simulink library "motohawk_engine_lib"  (Simulink 6.3)
undefined symbols (not defined in the file or in its folder): cast_val, IndPowerMax, InjSequence, lookup_group, MAF_Sensor_p, motohawk_tex, motohawk_vardec_config_group, motohawk_vardec_path, SampleTime, SparkSequence, SteadyStateECT, txtTitle, WarmUpTimeConst
libraries: MotoHawk_lib x234, motohawk_annotations_lib x22, motohawk_control_primitives_lib x20, motohawk_engine_lib x8, motohawk_control_primitives_lib_new x3
(part 2 of 7)

== system motohawk_engine_lib/Analog Switch ==
  ADC : Inport
  0 = No Inversion 1 = Inversion : MotoHawk_lib/Calibration & Probing Blocks/motohawk_calibration  nam=[prefix 'Polarity']  val=boolean(polarity-1)  storage=Calibration  show_more=on  name_source=Use Parameter  data_type=Inherit from 'Default Value'  read_level=1  write_level=1  ovr_cals=on  view_as=Number  enum_struct={'Disabled', 'Enabled'}  vector_style=Wide Row  use_help_units=on  help="'0 = High True    1 = Low True'"  units='bool'  use_header_enum=off  row_header_enum={}  col_header_enum={}  use_min_max=off  min_val=-inf  max_val=inf  use_precision=off  precision=''  gain=1  offset=0  exp=1  use_mototune_group=on  mototune_group=[group ' | ' nam ' Config']
  Data Type Conversion : DataTypeConversion  SaturateOnIntegerOverflow=on  RndMeth=Zero
  Logical Operator : Logic  Operator=XOR
  Override in Engineering Units : MotoHawk_lib/Calibration & Probing Blocks/motohawk_override_abs  parent_name=nam  show_more=on  name_source=Use Parameter  parent_read_level=1  parent_override_level=1  view_as=Number  enum_struct={'Disabled', 'Enabled'}  use_help_units=on  parent_help='Override actuator, in engineering units'  parent_units='Boolean'  use_min_max=off  parent_min=-inf  parent_max=inf  use_precision=off  parent_precision=''  parent_gain=1  parent_offset=0  parent_exp=1  use_mototune_group=on  parent_group=group
  Relational Operator : RelationalOperator  Operator=>
  SwitchPoint : MotoHawk_lib/Calibration & Probing Blocks/motohawk_calibration  nam=[prefix 'SwitchPt']  val=switchpoint  storage=Calibration  show_more=on  name_source=Use Parameter  data_type=Inherit from 'Default Value'  read_level=1  write_level=1  ovr_cals=on  view_as=Number  enum_struct={'Disabled', 'Enabled'}  vector_style=Wide Row  use_help_units=on  help='Defines switch point in ADC units boolean conversion'  units='ADC'  use_header_enum=off  row_header_enum={}  col_header_enum={}  use_min_max=off  min_val=-inf  max_val=inf  use_precision=off  precision=''  gain=1  offset=0  exp=1  use_mototune_group=on  mototune_group=[group ' | ' nam ' Config']
  motohawk_probe : MotoHawk_lib/Calibration & Probing Blocks/motohawk_probe  nam=nam  show_more=on  name_source=Use Parameter  read_level=1  view_as=Number  enum_struct={'Disabled', 'Enabled'}  vector_style=Wide Row  use_help_units=on  help='Display output in engineering units'  units='Boolean'  use_header_enum=off  row_header_enum={}  col_header_enum={}  use_precision=off  precision=''  gain=1  offset=0  exp=1  use_mototune_group=on  mototune_group=group
  motohawk_probe1 : MotoHawk_lib/Calibration & Probing Blocks/motohawk_probe  nam=[nam '_Raw']  show_more=on  name_source=Use Parameter  read_level=1  view_as=Number  enum_struct={'Disabled', 'Enabled'}  vector_style=Wide Row  use_help_units=on  help='Display output in engineering units'  units='ADC'  use_header_enum=off  row_header_enum={}  col_header_enum={}  use_precision=off  precision=''  gain=1  offset=0  exp=1  use_mototune_group=on  mototune_group=group
  DiscOut : Outport
  wires:
  ADC/1 -> Data Type Conversion/1
  0 = No Inversion 1 = Inversion/1 -> Logical Operator/2
  Logical Operator/1 -> Override in Engineering Units/1
  Relational Operator/1 -> Logical Operator/1
  SwitchPoint/1 -> Relational Operator/2
  Override in Engineering Units/1 -> DiscOut/1, motohawk_probe/1
  Data Type Conversion/1 -> Relational Operator/1, motohawk_probe1/1

== system motohawk_engine_lib/Analog Switch1 ==
  Boolean : Inport
  0 = No Inversion 1 = Inversion : MotoHawk_lib/Calibration & Probing Blocks/motohawk_calibration  nam=[prefix 'Polarity']  val=boolean(polarity-1)  storage=Calibration  show_more=on  name_source=Use Parameter  data_type=Inherit from 'Default Value'  read_level=1  write_level=1  ovr_cals=on  view_as=Number  enum_struct={'Disabled', 'Enabled'}  vector_style=Wide Row  use_help_units=on  help="'0 = High True    1 = Low True'"  units='bool'  use_header_enum=off  row_header_enum={}  col_header_enum={}  use_min_max=off  min_val=-inf  max_val=inf  use_precision=off  precision=''  gain=1  offset=0  exp=1  use_mototune_group=on  mototune_group=[group ' | ' nam ' Config']
  Logical Operator : Logic  Operator=XOR
  Override in Engineering Units : MotoHawk_lib/Calibration & Probing Blocks/motohawk_override_abs  parent_name=nam  show_more=on  name_source=Use Parameter  parent_read_level=1  parent_override_level=1  view_as=Number  enum_struct={'Disabled', 'Enabled'}  use_help_units=on  parent_help='Override actuator, in engineering units'  parent_units='Boolean'  use_min_max=off  parent_min=-inf  parent_max=inf  use_precision=off  parent_precision=''  parent_gain=1  parent_offset=0  parent_exp=1  use_mototune_group=on  parent_group=group
  motohawk_probe : MotoHawk_lib/Calibration & Probing Blocks/motohawk_probe  nam=nam  show_more=on  name_source=Use Parameter  read_level=1  view_as=Number  enum_struct={'Disabled', 'Enabled'}  vector_style=Wide Row  use_help_units=on  help='Display output in engineering units'  units='Boolean'  use_header_enum=off  row_header_enum={}  col_header_enum={}  use_precision=off  precision=''  gain=1  offset=0  exp=1  use_mototune_group=on  mototune_group=group
  motohawk_probe1 : MotoHawk_lib/Calibration & Probing Blocks/motohawk_probe  nam=[nam '_Raw']  show_more=on  name_source=Use Parameter  read_level=1  view_as=Number  enum_struct={'Disabled', 'Enabled'}  vector_style=Wide Row  use_help_units=on  help='Display output in engineering units'  units='Boolean'  use_header_enum=off  row_header_enum={}  col_header_enum={}  use_precision=off  precision=''  gain=1  offset=0  exp=1  use_mototune_group=on  mototune_group=group
  DiscOut : Outport
  wires:
  Override in Engineering Units/1 -> motohawk_probe/1, DiscOut/1
  Logical Operator/1 -> Override in Engineering Units/1
  0 = No Inversion 1 = Inversion/1 -> Logical Operator/2
  Boolean/1 -> Logical Operator/1, motohawk_probe1/1

== system motohawk_engine_lib/Capture Signal At Startup ==
  note: Count up to "BARO_Count" samples
  Signal_In : Inport
  Enable : EnablePort
  Add : Sum  OutScaling=2^-10
  Add1 : Sum  Inputs=+-  OutScaling=2^-10
  Collect Average : Subsystem
  Constant : Constant  Value=int8(1)  SampleTime=-1
  Logical Operator : Logic  AllPortsSameDT=off  OutDataTypeMode=Boolean
  Relational Operator : RelationalOperator  Operator=<=
  Relational Operator1 : RelationalOperator  Operator=>
  Sum : Sum  Inputs=++|  InputSameDT=on
  Switch : Switch  Threshold=1  ZeroCross=off  InputSameDT=on
  TwoSampleBuffer ToIgnore : Constant  Value=2  SampleTime=-1
  Unit Delay : UnitDelay  Orientation=left  SampleTime=-1
  motohawk_TitleBlock : motohawk_annotations_lib/motohawk_TitleBlock  BlockType_='Mototron_Title_Block'  ttl='Capture Signal At Key Up\newline\rmAverage the first \bfCount\rm samples of the signal on startup, before locking value.'  copyright="'THE INFORMATION CONTAINED IN THIS\\newlineDRAWING IS THE SOLE PROPERTY OF\\newlineMOTOTRON.  ANY REPRODUCTION IN\\newline PART OR AS A WHOLE WITHOUT THE\\newlineWRITTEN PERMISSION OF MOTOTRON\\newline IS PROHIBITED.\\fontsize{16}\\rm\\copyright\\rm\\fontsize{10} 2005'"  address='\fontsize{22}\it\fontname{Arial Black}MotoTron Corporation \fontname{Arial}\fontsize{10}\newline505 Marion Road, Oshkosh, WI, 54901\newlinewww.mototron.com (734) 822-7700'  image_file='mh.jpg'  pretty_print=on  edit_text="strrep([get_param(bdroot, 'Description')  '\\rm\\newline'  get_param(gcs, 'Name')], '_', '\\_')"  edit_as=255
  motohawk_calibration : MotoHawk_lib/Calibration & Probing Blocks/motohawk_calibration  nam=[nam '_Count']  val=int8(count)  storage=Calibration  show_more=on  name_source=Use Parameter  data_type=Inherit from 'Default Value'  read_level=1  write_level=1  ovr_cals=on  view_as=Number  enum_struct={'Disabled', 'Enabled'}  vector_style=Wide Row  use_help_units=on  help='Number of samples to average at key-up to produce signal value'  units=''  use_header_enum=off  row_header_enum={}  col_header_enum={}  use_min_max=off  min_val=-inf  max_val=inf  use_precision=off  precision=''  gain=1  offset=0  exp=1  use_mototune_group=on  mototune_group=grp
  motohawk_override_rel : MotoHawk_lib/Calibration & Probing Blocks/motohawk_override_rel  parent_name=nam  show_more=on  name_source=Use Parameter  parent_read_level=1  parent_override_level=1  use_help_units=on  parent_help='Provides an override to the input by adding this amount to either the locked or running value'  parent_units=units  use_min_max=off  parent_min=-inf  parent_max=inf  use_precision=off  parent_precision=''  parent_gain=1  parent_offset=0  parent_exp=1  use_mototune_group=on  parent_group=grp
  motohawk_probe : MotoHawk_lib/Calibration & Probing Blocks/motohawk_probe  nam=nam  show_more=on  name_source=Use Parameter  read_level=1  view_as=Number  enum_struct={'Disabled', 'Enabled'}  vector_style=Wide Row  use_help_units=on  help=''  units=units  use_header_enum=off  row_header_enum={}  col_header_enum={}  use_precision=off  precision=''  gain=1  offset=0  exp=1  use_mototune_group=on  mototune_group=grp
  Signal_KeyUp : Outport
  wires:
  Add1/1 -> Collect Average/1(Count)
  Relational Operator1/1 -> Logical Operator/2
  Logical Operator/1 -> Collect Average/Enable
  TwoSampleBuffer ToIgnore/1 -> Add1/2, Relational Operator1/2, Add/2
  Add/1 -> Switch/3, Relational Operator/2
  motohawk_calibration/1 -> Add/1
  motohawk_override_rel/1 -> Signal_KeyUp/1, motohawk_probe/1
  Constant/1 -> Sum/2
  Unit Delay/1 -> Sum/1
  Signal_In/1 -> Collect Average/2(Signal)
  Collect Average/1(Captured_Signal) -> motohawk_override_rel/1
  Switch/1 -> Add1/1, Unit Delay/1
  Relational Operator/1 -> Logical Operator/1, Switch/2
  Sum/1 -> Relational Operator1/1, Relational Operator/1, Switch/1

== system motohawk_engine_lib/Closed-Loop O2 Control - Dual Bank ==
  DesEquivRatio : Inport
  O2A [ratio] : Inport  Port=2
  O2B [ratio] : Inport  Port=3
  IndWork [kJ] : Inport  Port=4
  ClosedLoopEnable : Inport  Port=5
  Bus Creator : BusCreator  Inputs=3
  Map O2 Sensors to V8 Cylinders : Subsystem
      mask Display: disp('');
  Multiport Switch : MultiPortSwitch  Inputs=2  zeroidx=on  SaturateOnIntegerOverflow=on  InputSameDT=on
  No Multiplier When Disabled : Constant
  O2 Control State Determination : Subsystem
  O2A : motohawk_engine_lib/O2A  bank=A  display_group=lookup_group(gcb, 'O2Display')  cal_group=lookup_group(gcb, 'O2BankA')
  O2B : motohawk_engine_lib/O2A  bank=B  display_group=lookup_group(gcb, 'O2Display')  cal_group=lookup_group(gcb, 'O2BankB')
  motohawk_TitleBlock : motohawk_annotations_lib/motohawk_TitleBlock  BlockType_='Mototron_Title_Block'  ttl=[txtTitle '\newline\rmClosed-Loop O2 Control Algorithm']  copyright="'THE INFORMATION CONTAINED IN THIS\\newlineDRAWING IS THE SOLE PROPERTY OF\\newlineMOTOTRON.  ANY REPRODUCTION IN\\newline PART OR AS A WHOLE WITHOUT THE\\newlineWRITTEN PERMISSION OF MOTOTRON\\newline IS PROHIBITED.\\fontsize{16}\\rm\\copyright\\rm\\fontsize{10} 2005'"  address='\fontsize{22}\it\fontname{Arial Black}MotoTron Corporation \fontname{Arial}\fontsize{10}\newline505 Marion Road, Oshkosh, WI, 54901\newlinewww.mototron.com (734) 822-7700'  image_file='mh.jpg'  pretty_print=on  edit_text=[motohawk_tex(get_param(bdroot, 'Description')) '\rm\newline' motohawk_tex(get_param(gcs, 'Name'))]  edit_as=6
  motohawk_fault_action : MotoHawk_lib/Fault Management Blocks/motohawk_fault_action  nam='DisableO2Control'  eval_nam=DisableO2Control
  motohawk_probe : MotoHawk_lib/Calibration & Probing Blocks/motohawk_probe  nam='O2FuelMult'  show_more=on  name_source=Use Parameter  read_level=1  view_as=Number  enum_struct={'Disabled', 'Enabled'}  vector_style=Wide Row  use_help_units=on  help='Per-cylinder fuel multiplier for closed-loop O2 control'  units='mult'  use_header_enum=off  row_header_enum={}  col_header_enum={}  use_precision=off  precision=''  gain=1  offset=0  exp=1  use_mototune_group=on  mototune_group=lookup_group(gcb, 'O2Display')
  O2FuelMultVector : Outport
  O2Error : Outport  Port=2
  O2CtrlEnable : Outport  Port=3
  DesiredEqRatio : Outport  Port=4
  wires:
  O2 Control State Determination/1(O2Control) -> Multiport Switch/1, O2CtrlEnable/1, O2A/Enable, O2B/Enable
  No Multiplier When Disabled/1 -> Multiport Switch/2
  ClosedLoopEnable/1 -> O2 Control State Determination/1(O2ControlEnable [bool])
  Multiport Switch/1 -> motohawk_probe/1, O2FuelMultVector/1
  O2A [ratio]/1 -> O2A/1
  motohawk_fault_action/1 -> O2 Control State Determination/4(O2 Sensor Fault)
  IndWork [kJ]/1 -> O2 Control State Determination/3(IndWork [kJ])
  DesEquivRatio/1 -> DesiredEqRatio/1, O2 Control State Determination/2(DesEquivRatio), O2A/2, O2B/2
  O2B [ratio]/1 -> O2B/1
  Map O2 Sensors to V8 Cylinders/1(O2FuelMult [per-cylinder]) -> Multiport Switch/3
  O2A/1 -> Map O2 Sensors to V8 Cylinders/1(O2FuelMultA)
  O2B/1 -> Map O2 Sensors to V8 Cylinders/2(O2FuelMultB)
  Bus Creator/1 -> O2Error/1
  Map O2 Sensors to V8 Cylinders/2(BankCylSelectCal) -> Bus Creator/1  "CylSelectCals"
  O2A/2 -> Bus Creator/2  "BankA"
  O2B/2 -> Bus Creator/3  "BankB"

== system motohawk_engine_lib/Closed-Loop O2 Control - Single Bank ==
  DesEquivRatio : Inport
  O2A [ratio] : Inport  Port=2
  IndWork [kJ] : Inport  Port=3
  ClosedLoopEnable : Inport  Port=4
  Multiport Switch : MultiPortSwitch  Inputs=2  zeroidx=on  SaturateOnIntegerOverflow=on  InputSameDT=on
  No Multiplier When Disabled : Constant
  O2 Control State Determination : Subsystem
  O2A : motohawk_engine_lib/O2A  bank=A  display_group=lookup_group(gcb, 'O2Display')  cal_group=lookup_group(gcb, 'O2BankA')
  motohawk_TitleBlock : motohawk_annotations_lib/motohawk_TitleBlock  BlockType_='Mototron_Title_Block'  ttl=[txtTitle '\newline\rmClosed-Loop O2 Control Algorithm']  copyright="'THE INFORMATION CONTAINED IN THIS\\newlineDRAWING IS THE SOLE PROPERTY OF\\newlineMOTOTRON.  ANY REPRODUCTION IN\\newline PART OR AS A WHOLE WITHOUT THE\\newlineWRITTEN PERMISSION OF MOTOTRON\\newline IS PROHIBITED.\\fontsize{16}\\rm\\copyright\\rm\\fontsize{10} 2005'"  address='\fontsize{22}\it\fontname{Arial Black}MotoTron Corporation \fontname{Arial}\fontsize{10}\newline505 Marion Road, Oshkosh, WI, 54901\newlinewww.mototron.com (734) 822-7700'  image_file='mh.jpg'  pretty_print=on  edit_text=[motohawk_tex(get_param(bdroot, 'Description')) '\rm\newline' motohawk_tex(get_param(gcs, 'Name'))]  edit_as=6
  motohawk_fault_action : MotoHawk_lib/Fault Management Blocks/motohawk_fault_action  nam='DisableO2Control'  eval_nam=DisableO2Control
  motohawk_probe : MotoHawk_lib/Calibration & Probing Blocks/motohawk_probe  nam='O2FuelMult'  show_more=on  name_source=Use Parameter  read_level=1  view_as=Number  enum_struct={'Disabled', 'Enabled'}  vector_style=Wide Row  use_help_units=on  help='Per-cylinder fuel multiplier for closed-loop O2 control'  units='mult'  use_header_enum=off  row_header_enum={}  col_header_enum={}  use_precision=off  precision=''  gain=1  offset=0  exp=1  use_mototune_group=on  mototune_group='Engine Control | Run | O2 Control'
  O2FuelMult : Outport
  O2Error : Outport  Port=2
  O2CtrlEnable : Outport  Port=3
  DesiredEqRatio : Outport  Port=4
  wires:
  DesEquivRatio/1 -> O2 Control State Determination/2(DesEquivRatio), DesiredEqRatio/1, O2A/2
  IndWork [kJ]/1 -> O2 Control State Determination/3(IndWork [kJ])
  motohawk_fault_action/1 -> O2 Control State Determination/4(O2 Sensor Fault)
  O2A [ratio]/1 -> O2A/1
  O2A/1 -> Multiport Switch/3
  Multiport Switch/1 -> O2FuelMult/1, motohawk_probe/1
  ClosedLoopEnable/1 -> O2 Control State Determination/1(O2ControlEnable [bool])
  No Multiplier When Disabled/1 -> Multiport Switch/2
  O2 Control State Determination/1(O2Control) -> O2CtrlEnable/1, Multiport Switch/1, O2A/Enable
  O2A/2 -> O2Error/1

== system motohawk_engine_lib/Crank Synchronous SIgnal ==
  Signal_Time : Inport
  Merge : Merge
  Mux : Mux  Orientation=down  Inputs=2
  Once at Startup : Subsystem  TreatAsAtomicUnit=on
  TDC and MID_TDC : Subsystem  TreatAsAtomicUnit=on
  motohawk_trigger : MotoHawk_lib/Trigger Blocks/motohawk_trigger  Tag=Trigger  Orientation=down  trigger=FGND_TDC_EVENT  priority_order=0  inherited=off  run_disabled=off  override_app_monitor=off  target=ECU555_80
  motohawk_trigger1 : MotoHawk_lib/Trigger Blocks/motohawk_trigger  Tag=Trigger  Orientation=down  trigger=FGND_MID_TDC_EVENT  priority_order=0  inherited=off  run_disabled=off  override_app_monitor=off  target=ECU555_80
  motohawk_trigger2 : MotoHawk_lib/Trigger Blocks/motohawk_trigger  Tag=Trigger  Orientation=down  trigger=STARTUP_EVENT  priority_order=0  inherited=off  run_disabled=off  override_app_monitor=off  target=ECU555_80
  Signal_CA : Outport
  wires:
  TDC and MID_TDC/1(Signal_Ave) -> Merge/2
  Once at Startup/1(Signal_StartUp) -> Merge/1
  Merge/1 -> Signal_CA/1
  motohawk_trigger2/1 -> Once at Startup/Trigger
  motohawk_trigger1/1 -> Mux/2
  motohawk_trigger/1 -> Mux/1
  Mux/1 -> TDC and MID_TDC/Trigger
  Signal_Time/1 -> Once at Startup/1(Signal_Time), TDC and MID_TDC/1(Signal_Time)

== system motohawk_engine_lib/Discrete Actuator Characterization ==
  EngUnits : Inport
  0 = No Inversion 1 = Inversion : MotoHawk_lib/Calibration & Probing Blocks/motohawk_calibration  nam=[prefix '_Polarity']  val=boolean(polarity-1)  storage=Calibration  show_more=on  name_source=Use Parameter  data_type=Inherit from 'Default Value'  read_level=1  write_level=1  ovr_cals=on  view_as=Number  enum_struct={'Disabled', 'Enabled'}  vector_style=Wide Row  use_help_units=on  help="'Inverts the output of the actuator relative to the desired command - 0 = High True    1 = Low True'"  units='bool'  use_header_enum=off  row_header_enum={}  col_header_enum={}  use_min_max=off  min_val=-inf  max_val=inf  use_precision=off  precision=''  gain=1  offset=0  exp=1  use_mototune_group=on  mototune_group=[group ' | ' nam ' Config']
  Logical Operator : Logic  Operator=XOR
  Override in Engineering Units : MotoHawk_lib/Calibration & Probing Blocks/motohawk_override_abs  parent_name=prefix  show_more=on  name_source=Use Parameter  parent_read_level=1  parent_override_level=1  view_as=Number  enum_struct={'Disabled', 'Enabled'}  use_help_units=on  parent_help='Override actuator, in engineering units'  parent_units=units  use_min_max=off  parent_min=-inf  parent_max=inf  use_precision=off  parent_precision=''  parent_gain=1  parent_offset=0  parent_exp=1  use_mototune_group=on  parent_group=group
  Signal Specification : SignalSpecification  DataType=boolean
  motohawk_probe : MotoHawk_lib/Calibration & Probing Blocks/motohawk_probe  nam=prefix  show_more=on  name_source=Use Parameter  read_level=1  view_as=Number  enum_struct={'Disabled', 'Enabled'}  vector_style=Wide Row  use_help_units=on  help='Display output in engineering units'  units=units  use_header_enum=off  row_header_enum={}  col_header_enum={}  use_precision=off  precision=''  gain=1  offset=0  exp=1  use_mototune_group=on  mototune_group=group
  DiscOut : Outport
  wires:
  EngUnits/1 -> Signal Specification/1
  Signal Specification/1 -> Override in Engineering Units/1
  Override in Engineering Units/1 -> Logical Operator/1
  0 = No Inversion 1 = Inversion/1 -> Logical Operator/2
  Logical Operator/1 -> DiscOut/1, motohawk_probe/1

== system motohawk_engine_lib/Engine Steady-State Flag ==
  Load : Inport
  RPM : Inport  Port=2
  Abs : Abs  SaturateOnIntegerOverflow=on
  Abs1 : Abs  SaturateOnIntegerOverflow=on
  Constant : Constant  Value=0
  Filter IndTorque : motohawk_control_primitives_lib/First Order Low Pass (Tunable)  nam='SSLoadFiltConst'  time_const=.005  samp_time=samp_time  group=motohawk_vardec_config_group(group)
  Filter RPM : motohawk_control_primitives_lib/First Order Low Pass (Tunable)  nam='SSRPMFiltConst'  time_const=.005  samp_time=samp_time  group=motohawk_vardec_config_group(group)
  Logical Operator : Logic  Inputs=3
  Relational Operator : RelationalOperator  Operator=<=  InputSameDT=on
  Relational Operator1 : RelationalOperator  Operator=<=  InputSameDT=on
  Relational Operator2 : RelationalOperator  Operator=>  ZeroCross=off  InputSameDT=on
  Steady-state RPM Tolerance [RPM] : MotoHawk_lib/Calibration & Probing Blocks/motohawk_calibration  nam='SSRPMTol'  val=500  storage=Calibration  show_more=on  name_source=Use Parameter  data_type=Inherit from 'Default Value'  read_level=1  write_level=1  ovr_cals=on  view_as=Number  enum_struct={'Disabled', 'Enabled'}  vector_style=Wide Row  use_help_units=on  help='Steady-State RPM Tolerance'  units='RPM'  use_header_enum=off  row_header_enum={}  col_header_enum={}  use_min_max=off  min_val=-inf  max_val=inf  use_precision=off  precision=''  gain=1  offset=0  exp=1  use_mototune_group=on  mototune_group=motohawk_vardec_config_group(group)
  Steady-state Torque Tolerance [N.m] : MotoHawk_lib/Calibration & Probing Blocks/motohawk_calibration  nam='SSLoadTol'  val=50  storage=Calibration  show_more=on  name_source=Use Parameter  data_type=Inherit from 'Default Value'  read_level=1  write_level=1  ovr_cals=on  view_as=Number  enum_struct={'Disabled', 'Enabled'}  vector_style=Wide Row  use_help_units=on  help='Steady-State Load Tolerance'  units=''  use_header_enum=off  row_header_enum={}  col_header_enum={}  use_min_max=off  min_val=-inf  max_val=inf  use_precision=off  precision=''  gain=1  offset=0  exp=1  use_mototune_group=on  mototune_group=motohawk_vardec_config_group(group)
  Sum : Sum  Inputs=+-|  SaturateOnIntegerOverflow=on  InputSameDT=on
  Sum1 : Sum  Inputs=+-|  SaturateOnIntegerOverflow=on  InputSameDT=on
  motohawk_TitleBlock : motohawk_annotations_lib/motohawk_TitleBlock  BlockType_='Mototron_Title_Block'  ttl='Determine If the Engine is in Steady-State\newline\rmCheck whether the rates of change of RPM and Torque are slower than a threshold\newlineRPM must be nonzero for the engine to be steady-state'  copyright="'THE INFORMATION CONTAINED IN THIS\\newlineDRAWING IS THE SOLE PROPERTY OF\\newlineMOTOTRON.  ANY REPRODUCTION IN\\newline PART OR AS A WHOLE WITHOUT THE\\newlineWRITTEN PERMISSION OF MOTOTRON\\newline IS PROHIBITED.\\fontsize{16}\\rm\\copyright\\rm\\fontsize{10} 2005'"  address='\fontsize{22}\it\fontname{Arial Black}MotoTron Corporation \fontname{Arial}\fontsize{10}\newline505 Marion Road, Oshkosh, WI, 54901\newlinewww.mototron.com (734) 822-7700'  image_file='mh.jpg'  pretty_print=on  edit_text="strrep([get_param(bdroot, 'Description')  '\\rm\\newline'  get_param(gcs, 'Name')], '_', '\\_')"  edit_as=255
  motohawk_probe : MotoHawk_lib/Calibration & Probing Blocks/motohawk_probe  nam='SSEngOpr'  show_more=on  name_source=Use Parameter  read_level=1  view_as=Enumeration  enum_struct={'Transient', 'Steady'}  vector_style=Wide Row  use_help_units=on  help='Steady-State Engine Operation'  units=''  use_header_enum=off  row_header_enum={}  col_header_enum={}  use_precision=off  precision=''  gain=1  offset=0  exp=1  use_mototune_group=on  mototune_group=group
  SSEngOpr [bool] : Outport
  wires:
  Constant/1 -> Relational Operator2/2
  Relational Operator2/1 -> Logical Operator/2
  Relational Operator/1 -> Logical Operator/3
  Relational Operator1/1 -> Logical Operator/1
  Load/1 -> Filter IndTorque/1, Sum/1
  RPM/1 -> Relational Operator2/1, Filter RPM/1, Sum1/1
  Filter IndTorque/1 -> Sum/2
  Sum/1 -> Abs/1
  Abs/1 -> Relational Operator/1
  Sum1/1 -> Abs1/1
  Abs1/1 -> Relational Operator1/1
  Logical Operator/1 -> motohawk_probe/1, SSEngOpr [bool]/1
  Filter RPM/1 -> Sum1/2
  Steady-state Torque Tolerance [N.m]/1 -> Relational Operator/2
  Steady-state RPM Tolerance [RPM]/1 -> Relational Operator1/2

== system motohawk_engine_lib/Fuel Injector Output ==
  CylEnable : Inport
  Injector Common : Inport  Port=2
  Mechanical Pulse Width : Inport  Port=3
  Bus Selector : BusSelector  OutputSignals=Enable,SOI,PeakEPW,InjEPWOffset,EOI,MakeupMin
  Data Type Conversion{1..6} (6 alike) : DataTypeConversion  SaturateOnIntegerOverflow=on  RndMeth=Zero
  Gain{1,3..4,6} (4 alike) : Gain  Gain=1000  SaturateOnIntegerOverflow=on
  Gain2 : Gain  Gain=16  SaturateOnIntegerOverflow=on
  Gain5 : Gain  Gain=16  SaturateOnIntegerOverflow=on
  Logical Operator : Logic  AllPortsSameDT=off
  motohawk_injector : MotoHawk_lib/Advanced Digital I//O/motohawk_injector  text_resource=FINJ1  code_resource=RES_INJ1D  val_resource=-1  target=ECU555_80  resource_enum_str=(None)=-1,FINJ1=12,FINJ2=13,FINJ3=14,FINJ4=15,FINJ5=16,FINJ6=17,FINJ7=18,AINJ1=18,FINJ8=19,AINJ2=19,FINJ9=20,AINJ3=20,FINJ10=21,AINJ4=21,FINJ11=22,AINJ5=22,FINJ12=23,AINJ6=23  behavior=Transient  update_mode=OS  granularity=Fine  angle_offset=offset  min_eoi_soi_angle=90  use_vardec=off  nam='INJ'  read_level=1  write_level=1  group='System | I/O Pins | Outputs Config'
  wires:
  Bus Selector/2 -> Gain2/1  "<SOI>"
  Bus Selector/5 -> Gain5/1  "<EOI>"
  Mechanical Pulse Width/1 -> Gain1/1
  Bus Selector/3 -> Gain4/1  "<PeakEPW>"
  Bus Selector/6 -> Gain6/1  "<MakeupMin>"
  Gain3/1 -> Data Type Conversion3/1
  Bus Selector/4 -> Gain3/1  "<InjEPWOffset>"
  Gain2/1 -> Data Type Conversion1/1
  Gain1/1 -> Data Type Conversion2/1
  Gain4/1 -> Data Type Conversion4/1
  Injector Common/1 -> Bus Selector/1
  Gain5/1 -> Data Type Conversion5/1
  Gain6/1 -> Data Type Conversion6/1
  Data Type Conversion1/1 -> motohawk_injector/2
  Data Type Conversion4/1 -> motohawk_injector/4
  Data Type Conversion3/1 -> motohawk_injector/5
  Data Type Conversion6/1 -> motohawk_injector/7
  Data Type Conversion2/1 -> motohawk_injector/3
  Data Type Conversion5/1 -> motohawk_injector/6
  Logical Operator/1 -> motohawk_injector/1
  Bus Selector/1 -> Logical Operator/2  "<Enable>"
  CylEnable/1 -> Logical Operator/1

== system motohawk_engine_lib/Idle Governor ==
  RPM : Inport
  ECT [C] : Inport  Port=2
  ThrPos [%] : Inport  Port=3
  Idle State Determination : Subsystem
      mask Display: disp('IDLE STATE\nDETERMINATION');
  Logical Operator : Logic  Operator=NOT
  Ramp RPM : Subsystem
      mask Display: disp('RAMP RPM\nINTO IDLE STATE');
  Terminator3 : Terminator
  Universal PD (Tunable) : motohawk_control_primitives_lib/Universal PD (Tunable)  nam='Idle Spark Control'  prefix='IdleSpark_'  DCOffset=0  PGain=3  DGain=0  ErrorGain=1.0  OutLwrLim=-10  OutUprLim=20  samp_time=SampleTime  units=''  group=motohawk_vardec_path(gcb)
  Universal PID (Tunable) : motohawk_control_primitives_lib/Universal PID (Tunable)  nam='Idle Air Control'  prefix='IdleAir_'  DCOffset=0  PGain=0  IGain=20  DGain=0  ErrorGain=1.0  ITermLwrLim=0  ITermUprLim=100  OutLwrLim=0  OutUprLim=100  samp_time=SampleTime  units=''  group=motohawk_vardec_path(gcb)
  motohawk_TitleBlock : motohawk_annotations_lib/motohawk_TitleBlock  BlockType_='Mototron_Title_Block'  ttl='Idle RPM Governor'  copyright="'THE INFORMATION CONTAINED IN THIS\\newlineDRAWING IS THE SOLE PROPERTY OF\\newlineMOTOTRON.  ANY REPRODUCTION IN\\newline PART OR AS A WHOLE WITHOUT THE\\newlineWRITTEN PERMISSION OF MOTOTRON\\newline IS PROHIBITED.\\fontsize{16}\\rm\\copyright\\rm\\fontsize{10} 2005'"  address='\fontsize{22}\it\fontname{Arial Black}MotoTron Corporation \fontname{Arial}\fontsize{10}\newline505 Marion Road, Oshkosh, WI, 54901\newlinewww.mototron.com (734) 822-7700'  image_file='mh.jpg'  pretty_print=on  edit_text=[motohawk_tex(get_param(bdroot, 'Description')) '\rm\newline' motohawk_tex(get_param(gcs, 'Name'))]  edit_as=6
  motohawk_calibration2 : MotoHawk_lib/Calibration & Probing Blocks/motohawk_calibration  nam='IdleTargetRPM'  val=500  storage=Calibration  show_more=on  name_source=Use Parameter  data_type=Inherit from 'Default Value'  read_level=1  write_level=1  ovr_cals=on  view_as=Number  enum_struct={'Disabled', 'Enabled'}  vector_style=Wide Row  use_help_units=off  help=''  units=''  use_header_enum=off  row_header_enum={}  col_header_enum={}  use_min_max=off  min_val=-inf  max_val=inf  use_precision=off  precision=''  gain=1  offset=0  exp=1  use_mototune_group=off  mototune_group=motohawk_vardec_path(gcb)
  SparkAdv Offset [degCA] : Outport
  LIAC Offset [%] : Outport  Port=2
  wires:
  Logical Operator/1 -> Universal PID (Tunable)/3
  motohawk_calibration2/1 -> Ramp RPM/3(TargetRPM), Idle State Determination/2(TargetRPM)
  Universal PID (Tunable)/1 -> LIAC Offset [%]/1
  Idle State Determination/1(OnIdle) -> Logical Operator/1, Ramp RPM/1(OnIdle)
  Ramp RPM/1(RPMSetPt) -> Universal PD (Tunable)/2, Universal PID (Tunable)/2  "RPMSetPt"
  Universal PD (Tunable)/1 -> SparkAdv Offset [degCA]/1
  ThrPos [%]/1 -> Idle State Determination/3(ThrPos [%])
  RPM/1 -> Universal PID (Tunable)/1, Universal PD (Tunable)/1, Ramp RPM/2(RPM), Idle State Determination/1(RPM)  "RPM"
  ECT [C]/1 -> Terminator3/1

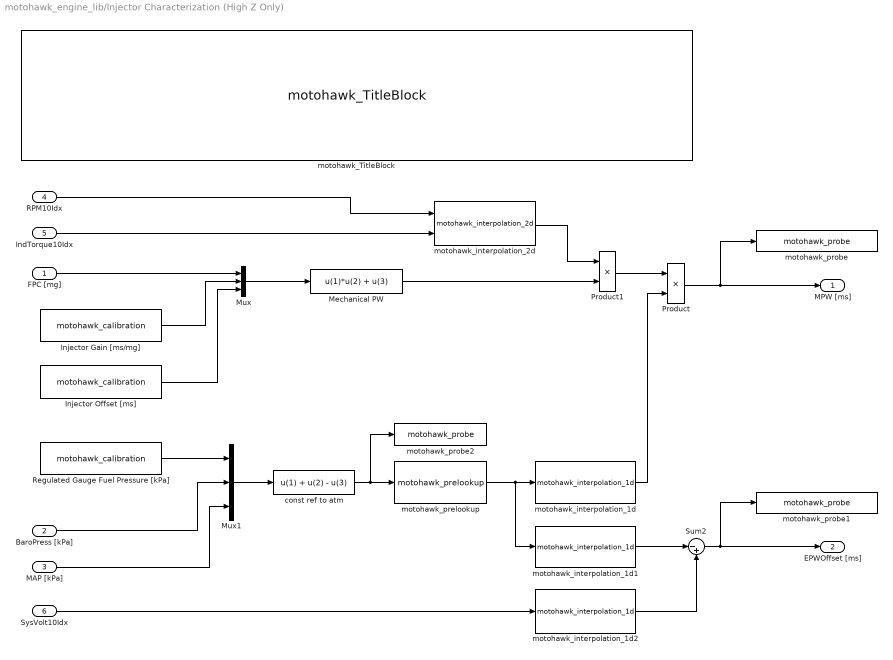
== system motohawk_engine_lib/Injector Characterization (High Z Only) ==
  FPC [mg] : Inport
  BaroPress [kPa] : Inport  Port=2
  MAP [kPa] : Inport  Port=3
  RPM10Idx : Inport  Port=4
  IndTorque10Idx : Inport  Port=5
  SysVolt10Idx : Inport  Port=6
  Injector Gain [ms/mg] : MotoHawk_lib/Calibration & Probing Blocks/motohawk_calibration  nam='InjGain'  val=InjGain  storage=Calibration  show_more=on  name_source=Use Parameter  data_type=Inherit from 'Default Value'  read_level=1  write_level=1  ovr_cals=on  view_as=Number  enum_struct={'Disabled', 'Enabled'}  vector_style=Wide Row  use_help_units=on  help='Injector Gain - FPC to MPW'  units='ms/mg'  use_header_enum=off  row_header_enum={}  col_header_enum={}  use_min_max=off  min_val=-inf  max_val=inf  use_precision=off  precision=''  gain=1  offset=0  exp=1  use_mototune_group=off  mototune_group=lookup_group(gcb, 'InjGain')
  Injector Offset [ms] : MotoHawk_lib/Calibration & Probing Blocks/motohawk_calibration  nam='InjOffset'  val=InjOffset  storage=Calibration  show_more=on  name_source=Use Parameter  data_type=Inherit from 'Default Value'  read_level=1  write_level=1  ovr_cals=on  view_as=Number  enum_struct={'Disabled', 'Enabled'}  vector_style=Wide Row  use_help_units=on  help='Injector Offset - FPC to MPW'  units='ms'  use_header_enum=off  row_header_enum={}  col_header_enum={}  use_min_max=off  min_val=-inf  max_val=inf  use_precision=off  precision=''  gain=1  offset=0  exp=1  use_mototune_group=off  mototune_group=lookup_group(gcb, 'InjOffset')
  Mechanical PW : Fcn  Expr=u(1)*u(2) + u(3)
  Mux : Mux  Inputs=3
  Mux1 : Mux  Inputs=3
  Product : Product  SaturateOnIntegerOverflow=on
  Product1 : Product  SaturateOnIntegerOverflow=on
  Regulated Gauge Fuel Pressure [kPa] : MotoHawk_lib/Calibration & Probing Blocks/motohawk_calibration  nam='GaugeFuelPress'  val=GaugeFuelPress  storage=Calibration  show_more=on  name_source=Use Parameter  data_type=Inherit from 'Default Value'  read_level=1  write_level=1  ovr_cals=on  view_as=Number  enum_struct={'Disabled', 'Enabled'}  vector_style=Wide Row  use_help_units=on  help='Regulated Gauge Fuel Pressure'  units='kPa'  use_header_enum=off  row_header_enum={}  col_header_enum={}  use_min_max=off  min_val=-inf  max_val=inf  use_precision=off  precision=''  gain=1  offset=0  exp=1  use_mototune_group=off  mototune_group=lookup_group(gcb, 'GaugeFuelPress')
  Sum2 : Sum  Inputs=|-+  SaturateOnIntegerOverflow=on
  const ref to atm : Fcn  Expr=u(1) + u(2) - u(3)
  motohawk_TitleBlock : motohawk_annotations_lib/motohawk_TitleBlock  BlockType_='Mototron_Title_Block'  ttl='Fuel Injector Characterization\newline\rmCalculations for High-Impedance Injectors'  copyright="'THE INFORMATION CONTAINED IN THIS\\newlineDRAWING IS THE SOLE PROPERTY OF\\newlineMOTOTRON.  ANY REPRODUCTION IN\\newline PART OR AS A WHOLE WITHOUT THE\\newlineWRITTEN PERMISSION OF MOTOTRON\\newline IS PROHIBITED.\\fontsize{16}\\rm\\copyright\\rm\\fontsize{10} 2005'"  address='\fontsize{22}\it\fontname{Arial Black}MotoTron Corporation \fontname{Arial}\fontsize{10}\newline505 Marion Road, Oshkosh, WI, 54901\newlinewww.mototron.com (734) 822-7700'  image_file='mh.jpg'  pretty_print=on  edit_text=[motohawk_tex(get_param(bdroot, 'Description')) '\rm\newline' motohawk_tex(get_param(gcs, 'Name'))]  edit_as=6
  motohawk_interpolation_1d : MotoHawk_lib/Lookup Tables/motohawk_interpolation_1d  nam='FueldPComp'  table_data=FueldPCompTbl  show_more=on  data_type=Inherit from 'Table Data'  storage=NonAdaptive  read_level=1  write_level=1  ovr_cals=on  use_help=on  help='Fuel Delta Pressure Compensation'  units='mult'  use_min_max=off  min_val=-inf  max_val=inf  use_precision=off  precision=''  gain=1  offset=0  exp=1  use_links=off  prelookup_block=''  output_name=''  use_mototune_group=off  mototune_group=lookup_group(gcb, 'FueldPComp')
  motohawk_interpolation_1d1 : MotoHawk_lib/Lookup Tables/motohawk_interpolation_1d  nam='InjTurnOff'  table_data=InjTurnOffTbl  show_more=on  data_type=Inherit from 'Table Data'  storage=NonAdaptive  read_level=1  write_level=1  ovr_cals=on  use_help=on  help='Injector Turn Off Time'  units='ms'  use_min_max=off  min_val=-inf  max_val=inf  use_precision=off  precision=''  gain=1  offset=0  exp=1  use_links=off  prelookup_block=''  output_name=''  use_mototune_group=off  mototune_group=lookup_group(gcb, 'InjTurnOff')
  motohawk_interpolation_1d2 : MotoHawk_lib/Lookup Tables/motohawk_interpolation_1d  nam='InjTurnOn'  table_data=InjTurnOnTbl  show_more=on  data_type=Inherit from 'Table Data'  storage=NonAdaptive  read_level=1  write_level=1  ovr_cals=on  use_help=on  help='Injector Turn On Time'  units='ms'  use_min_max=off  min_val=-inf  max_val=inf  use_precision=off  precision=''  gain=1  offset=0  exp=1  use_links=off  prelookup_block=''  output_name=''  use_mototune_group=off  mototune_group=lookup_group(gcb, 'InjTurnOn')
  motohawk_interpolation_2d : MotoHawk_lib/Lookup Tables/motohawk_interpolation_2d  nam='FuelFlowComp'  table_data=FuelFlowCompMap  show_more=on  data_type=Inherit from 'Table Data'  storage=NonAdaptive  read_level=1  write_level=1  ovr_cals=on  use_help=on  help='Fuel Flow Compensation Multiplier - gain to adjust mechanical injector pulse width'  units='mult'  use_min_max=off  min_val=-inf  max_val=inf  use_precision=off  precision=''  gain=1  offset=0  exp=1  use_links=off  row_prelookup_block=''  col_prelookup_block=''  output_name=''  use_mototune_group=off  mototune_group=lookup_group(gcb, 'FuelFlowComp')
  motohawk_prelookup : MotoHawk_lib/Lookup Tables/motohawk_prelookup  nam='FuelDeltaPress10'  breakpoint_data=FuelDeltaPress10IdxArr  show_more=on  data_type=Inherit from 'Table Data'  storage=Constant  read_level=1  write_level=1  ovr_cals=on  use_help=on  help='Fuel Delta Breakpoints'  units='kPa'  use_min_max=off  min_val=-inf  max_val=inf  use_precision=off  precision=''  gain=1  offset=0  exp=1  use_links=on  input_name='FuelDeltaPress'  use_mototune_group=off  mototune_group=lookup_group(gcb, 'FuelDeltaPress10')
  motohawk_probe : MotoHawk_lib/Calibration & Probing Blocks/motohawk_probe  nam='InjMPW'  show_more=on  name_source=Use Parameter  read_level=1  view_as=Number  enum_struct={'Disabled', 'Enabled'}  vector_style=Wide Row  use_help_units=on  help='Injector Mechanical Pulse Width'  units='ms'  use_header_enum=off  row_header_enum={}  col_header_enum={}  use_precision=off  precision=''  gain=1  offset=0  exp=1  use_mototune_group=off  mototune_group=lookup_group(gcb, 'InjMPW')
  motohawk_probe1 : MotoHawk_lib/Calibration & Probing Blocks/motohawk_probe  nam='InjEPWOffset'  show_more=on  name_source=Use Parameter  read_level=1  view_as=Number  enum_struct={'Disabled', 'Enabled'}  vector_style=Wide Row  use_help_units=on  help='Injector mechanical to electrical pulse width offset'  units='ms'  use_header_enum=off  row_header_enum={}  col_header_enum={}  use_precision=off  precision=''  gain=1  offset=0  exp=1  use_mototune_group=off  mototune_group=lookup_group(gcb, 'InjEPWOffset')
  motohawk_probe2 : MotoHawk_lib/Calibration & Probing Blocks/motohawk_probe  nam='FuelDeltaPress'  show_more=on  name_source=Use Parameter  read_level=1  view_as=Number  enum_struct={'Disabled', 'Enabled'}  vector_style=Wide Row  use_help_units=on  help='Fuel Delta Pressure - across the fuel injector'  units='kPa'  use_header_enum=off  row_header_enum={}  col_header_enum={}  use_precision=off  precision=''  gain=1  offset=0  exp=1  use_mototune_group=off  mototune_group=lookup_group(gcb, 'FuelDeltaPress')
  MPW [ms] : Outport
  EPWOffset [ms] : Outport  Port=2
  wires:
  IndTorque10Idx/1 -> motohawk_interpolation_2d/2
  motohawk_prelookup/1 -> motohawk_interpolation_1d/1, motohawk_interpolation_1d1/1
  FPC [mg]/1 -> Mux/1
  Mux/1 -> Mechanical PW/1
  Injector Gain [ms/mg]/1 -> Mux/2
  Injector Offset [ms]/1 -> Mux/3
  SysVolt10Idx/1 -> motohawk_interpolation_1d2/1
  Mechanical PW/1 -> Product1/2
  motohawk_interpolation_1d2/1 -> Sum2/2
  motohawk_interpolation_1d1/1 -> Sum2/1
  const ref to atm/1 -> motohawk_prelookup/1, motohawk_probe2/1
  Mux1/1 -> const ref to atm/1
  Regulated Gauge Fuel Pressure [kPa]/1 -> Mux1/1
  BaroPress [kPa]/1 -> Mux1/2
  MAP [kPa]/1 -> Mux1/3
  motohawk_interpolation_1d/1 -> Product/2
  Product/1 -> MPW [ms]/1, motohawk_probe/1
  Sum2/1 -> EPWOffset [ms]/1, motohawk_probe1/1
  Product1/1 -> Product/1
  motohawk_interpolation_2d/1 -> Product1/1
  RPM10Idx/1 -> motohawk_interpolation_2d/1

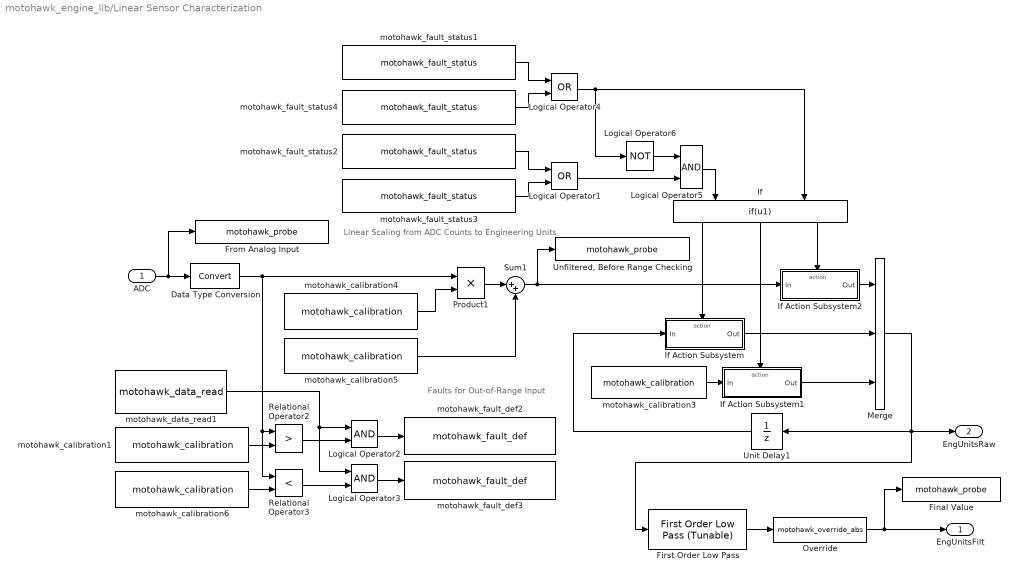
== system motohawk_engine_lib/Linear Sensor Characterization ==
  note: Faults for
      | Out-of-Range
      | Input
  note: Linear Scaling from ADC Counts
      | to Engineering Units
  ADC : Inport
  Data Type Conversion : DataTypeConversion  SaturateOnIntegerOverflow=on  RndMeth=Zero
  Final Value : MotoHawk_lib/Calibration & Probing Blocks/motohawk_probe  nam=nam  show_more=on  name_source=Use Parameter  read_level=1  view_as=Number  enum_struct={'Disabled', 'Enabled'}  vector_style=Wide Row  use_help_units=on  help='Final value after Linear Sensor Characterization'  units=units  use_header_enum=off  row_header_enum={}  col_header_enum={}  use_precision=off  precision=''  gain=1  offset=0  exp=1  use_mototune_group=on  mototune_group=group
  First Order Low Pass : motohawk_control_primitives_lib/First Order Low Pass (Tunable)  nam=[prefix 'FilterConst']  samp_time=samp_time  group=[group ' | ' nam ' Config']
  From Analog Input : MotoHawk_lib/Calibration & Probing Blocks/motohawk_probe  nam=[prefix 'ADC']  show_more=on  name_source=Use Parameter  read_level=1  view_as=Number  enum_struct={'Disabled', 'Enabled'}  vector_style=Wide Row  use_help_units=on  help='Singal measured directly from sensor'  units=inputunits  use_header_enum=off  row_header_enum={}  col_header_enum={}  use_precision=off  precision=''  gain=1  offset=0  exp=1  use_mototune_group=on  mototune_group=group
  If : If  Orientation=down  NumInputs=2  IfExpression=u1  ElseIfExpressions=u2  ZeroCross=off
  If Action Subsystem : Subsystem  TreatAsAtomicUnit=on
      mask Display: disp('Saturate');
  If Action Subsystem1 : Subsystem  TreatAsAtomicUnit=on
      mask Display: disp('Default');
  If Action Subsystem2 : Subsystem  TreatAsAtomicUnit=on
      mask Display: disp('Pass Through');
  Logical Operator1 : Logic  Operator=OR
  Logical Operator2 : Logic
  Logical Operator3 : Logic
  Logical Operator4 : Logic  Operator=OR
  Logical Operator5 : Logic
  Logical Operator6 : Logic  Operator=NOT
  Merge : Merge  Inputs=3
  Override : MotoHawk_lib/Calibration & Probing Blocks/motohawk_override_abs  parent_name=nam  show_more=on  name_source=Use Parameter  parent_read_level=1  parent_override_level=1  view_as=Number  enum_struct={'Disabled', 'Enabled'}  use_help_units=on  parent_help='Override result of linear sensor characterization, in engineering units'  parent_units=units  use_min_max=on  parent_min=-inf  parent_max=inf  use_precision=off  parent_precision=''  parent_gain=1  parent_offset=0  parent_exp=1  use_mototune_group=on  parent_group=group
  Product1 : Product  SaturateOnIntegerOverflow=on  InputSameDT=on
  Relational Operator2 : RelationalOperator  Operator=>  ZeroCross=off  InputSameDT=on
  Relational Operator3 : RelationalOperator  Operator=<  ZeroCross=off  InputSameDT=on
  Sum1 : Sum  Inputs=|++  SaturateOnIntegerOverflow=on
  "Unfiltered, Before Range Checking" : MotoHawk_lib/Calibration & Probing Blocks/motohawk_probe  nam=[prefix 'Raw']  show_more=on  name_source=Use Parameter  read_level=1  view_as=Number  enum_struct={'Disabled', 'Enabled'}  vector_style=Wide Row  use_help_units=on  help='After conversion to engineering units, before range checking'  units=units  use_header_enum=off  row_header_enum={}  col_header_enum={}  use_precision=off  precision=''  gain=1  offset=0  exp=1  use_mototune_group=on  mototune_group=group
  Unit Delay1 : UnitDelay  Orientation=left  SampleTime=-1
  motohawk_calibration1 : MotoHawk_lib/Calibration & Probing Blocks/motohawk_calibration  nam=[prefix 'InputHiFltPos']  val=1020  storage=Calibration  show_more=on  name_source=Use Parameter  data_type=double  read_level=1  write_level=1  ovr_cals=on  view_as=Number  enum_struct={'Disabled', 'Enabled'}  vector_style=Wide Row  use_help_units=on  help='Maximum allowable input, indicating short or open circuit'  units=inputunits  use_header_enum=off  row_header_enum={}  col_header_enum={}  use_min_max=off  min_val=-inf  max_val=inf  use_precision=off  precision=''  gain=1  offset=0  exp=1  use_mototune_group=on  mototune_group=[group ' | ' nam ' Config']
  motohawk_calibration3 : MotoHawk_lib/Calibration & Probing Blocks/motohawk_calibration  nam=[prefix 'DfltValue']  val=1  storage=Calibration  show_more=on  name_source=Use Parameter  data_type=double  read_level=1  write_level=1  ovr_cals=on  view_as=Number  enum_struct={'Disabled', 'Enabled'}  vector_style=Wide Row  use_help_units=on  help="'This is the initial default value should the sensor be in fault on key-up.  Otherwise the sensors outputs the last value prior to faulting'"  units=units  use_header_enum=off  row_header_enum={}  col_header_enum={}  use_min_max=off  min_val=-inf  max_val=inf  use_precision=off  precision=''  gain=1  offset=0  exp=1  use_mototune_group=on  mototune_group=[group ' | ' nam ' Config']
  motohawk_calibration4 : MotoHawk_lib/Calibration & Probing Blocks/motohawk_calibration  nam=[prefix 'Gain']  val=1  storage=Calibration  show_more=on  name_source=Use Parameter  data_type=double  read_level=1  write_level=1  ovr_cals=on  view_as=Number  enum_struct={'Disabled', 'Enabled'}  vector_style=Wide Row  use_help_units=on  help='Scaling from A/D counts to engineering units'  units=[units '/ADC']  use_header_enum=off  row_header_enum={}  col_header_enum={}  use_min_max=off  min_val=-inf  max_val=inf  use_precision=on  precision='5.4'  gain=1  offset=0  exp=1  use_mototune_group=on  mototune_group=[group ' | ' nam ' Config']
  motohawk_calibration5 : MotoHawk_lib/Calibration & Probing Blocks/motohawk_calibration  nam=[prefix 'Ofst']  val=0  storage=Calibration  show_more=on  name_source=Use Parameter  data_type=double  read_level=1  write_level=1  ovr_cals=on  view_as=Number  enum_struct={'Disabled', 'Enabled'}  vector_style=Wide Row  use_help_units=on  help='Offset after gain in engineering units'  units=units  use_header_enum=off  row_header_enum={}  col_header_enum={}  use_min_max=off  min_val=-inf  max_val=inf  use_precision=off  precision=''  gain=1  offset=0  exp=1  use_mototune_group=on  mototune_group=[group ' | ' nam ' Config']
  motohawk_calibration6 : MotoHawk_lib/Calibration & Probing Blocks/motohawk_calibration  nam=[prefix 'InputLoFltPos']  val=10  storage=Calibration  show_more=on  name_source=Use Parameter  data_type=double  read_level=1  write_level=1  ovr_cals=on  view_as=Number  enum_struct={'Disabled', 'Enabled'}  vector_style=Wide Row  use_help_units=on  help='Minimum allowable input, indicating short or open circuit'  units=inputunits  use_header_enum=off  row_header_enum={}  col_header_enum={}  use_min_max=off  min_val=-inf  max_val=inf  use_precision=off  precision=''  gain=1  offset=0  exp=1  use_mototune_group=on  mototune_group=[group ' | ' nam ' Config']
  motohawk_data_read1 : MotoHawk_lib/Data Storage Blocks/motohawk_data_read  source=Lookup By Name  structure=Scalar  operation=Read entire data structure at once  sz_vec=4  sz_row=2  sz_col=3  typ=boolean  nam='MPRD'  checkNull=on  struct_inst_name='Struct1'
  motohawk_fault_def2 : MotoHawk_lib/Fault Management Blocks/motohawk_fault_def  nam=[prefix 'RangeHigh']  mode=Enabled  id=[]  x=25  y=50  input_suspected=on  indeterminate=off  increment_xy=on  downsample_count=1  ovr_cals=on  ovr_actions=on  show_actions=off  action1_name=''  action1_cond=(None)  action2_name=''  action2_cond=(None)  action3_name=''  action3_cond=(None)  action4_name=''  action4_cond=(None)
  motohawk_fault_def3 : MotoHawk_lib/Fault Management Blocks/motohawk_fault_def  nam=[prefix 'RangeLow']  mode=Enabled  id=[]  x=25  y=50  input_suspected=on  indeterminate=off  increment_xy=on  downsample_count=1  ovr_cals=on  ovr_actions=on  show_actions=off  action1_name=''  action1_cond=(None)  action2_name=''  action2_cond=(None)  action3_name=''  action3_cond=(None)  action4_name=''  action4_cond=(None)
  motohawk_fault_status1 : MotoHawk_lib/Fault Management Blocks/motohawk_fault_status  source=Lookup By Name  nam=[prefix 'RangeHigh']  status=Active
  motohawk_fault_status2 : MotoHawk_lib/Fault Management Blocks/motohawk_fault_status  source=Lookup By Name  nam=[prefix 'RangeHigh']  status=Suspected
  motohawk_fault_status3 : MotoHawk_lib/Fault Management Blocks/motohawk_fault_status  source=Lookup By Name  nam=[prefix 'RangeLow']  status=Suspected
  motohawk_fault_status4 : MotoHawk_lib/Fault Management Blocks/motohawk_fault_status  source=Lookup By Name  nam=[prefix 'RangeLow']  status=Active
  EngUnitsFilt : Outport
  EngUnitsRaw : Outport  Port=2
  wires:
  Merge/1 -> Unit Delay1/1, EngUnitsRaw/1, First Order Low Pass/1
  If/3 -> If Action Subsystem2/Action
  If/1 -> If Action Subsystem/Action
  Data Type Conversion/1 -> Relational Operator2/1, Relational Operator3/1, Product1/1
  ADC/1 -> From Analog Input/1, Data Type Conversion/1
  Override/1 -> Final Value/1, EngUnitsFilt/1
  motohawk_calibration4/1 -> Product1/2
  motohawk_calibration5/1 -> Sum1/2
  Product1/1 -> Sum1/1
  motohawk_data_read1/1 -> Logical Operator2/1, Logical Operator3/1
  Logical Operator3/1 -> motohawk_fault_def3/1
  Logical Operator2/1 -> motohawk_fault_def2/1
  Relational Operator3/1 -> Logical Operator3/2
  Relational Operator2/1 -> Logical Operator2/2
  motohawk_calibration1/1 -> Relational Operator2/2
  motohawk_calibration6/1 -> Relational Operator3/2
  motohawk_fault_status2/1 -> Logical Operator1/1
  motohawk_fault_status3/1 -> Logical Operator1/2
  If Action Subsystem2/1(Out) -> Merge/1
  If Action Subsystem/1(Out) -> Merge/2
  Sum1/1 -> If Action Subsystem2/1(In), "Unfiltered, Before Range Checking"/1
  motohawk_fault_status1/1 -> Logical Operator4/1
  motohawk_fault_status4/1 -> Logical Operator4/2
  If Action Subsystem1/1(Out) -> Merge/3
  If/2 -> If Action Subsystem1/Action
  Unit Delay1/1 -> If Action Subsystem/1(In)
  motohawk_calibration3/1 -> If Action Subsystem1/1(In)
  First Order Low Pass/1 -> Override/1
  Logical Operator6/1 -> Logical Operator5/1
  Logical Operator5/1 -> If/1
  Logical Operator1/1 -> Logical Operator5/2
  Logical Operator4/1 -> Logical Operator6/1, If/2
